simulink model "tanqueNL"  (R2018b)
settings: Solver=VariableStepAuto  StartTime=0.0  StopTime=500  RelTol=1e-3
values from neighbouring files (symbols this model uses):
  A = A    [controleLQR.m]    (also in dadosTanque.m = ssT.A; tanqueSS.m = subs(A,{qin1,qin2,h1,h2},{qin1_barra,qin2_barra,h1_barra,h2_)
  B2 = B2    [controleLQR.m]    (also in dadosTanque.m = ssT.B)
  C = C    [controleLQR.m]    (also in dadosTanque.m = ssT.C; tanqueSS.m = [1 0;0 1])
  D = D    [controleLQR.m]    (also in dadosTanque.m = ssT.D; tanqueSS.m = [0 0;0 0])
  h1 = 25    [dadosTanque.m]    (also in filterTest.m = h1_ruido(1:end-1); frequencyAnalysis.m = h1_ruido(500:1200); ssTanque.m = h1_ruido(1:end-1))
  h2 = 20    [dadosTanque.m]    (also in ssTanque.m = h2_ruido(1:end-1))
  k1 = 25    [dadosTanque.m]    (also in tanqueSS.m)
  k2 = 25    [dadosTanque.m]    (also in tanqueSS.m)
  kac = 20    [dadosTanque.m]    (also in tanqueSS.m)
  qin1 = k1*sqrt(h1) + kac*sqrt(h1-h2)    [dadosTanque.m]    (also in dados_tanque.mat = [169.72135955 169.72135955 169.72135955 169.72135955 169.721)
  qin2 = k2*sqrt(h2) - kac*sqrt(h1-h2)    [dadosTanque.m]    (also in dados_tanque.mat = [67.082039325 67.082039325 67.082039325 67.082039325 67.0820)
  stepTime = 0    [comparacao_controle_graficos.m]    (also in comparacao_sistema_graficos.m = 20; dadosTanque.m = 100)
  stepValueh1 = 1    [comparacao_controle_graficos.m]    (also in comparacao_sistema_graficos.m; dadosTanque.m)
settings Model: Creator=Caléo  LastModifiedBy=Caléo

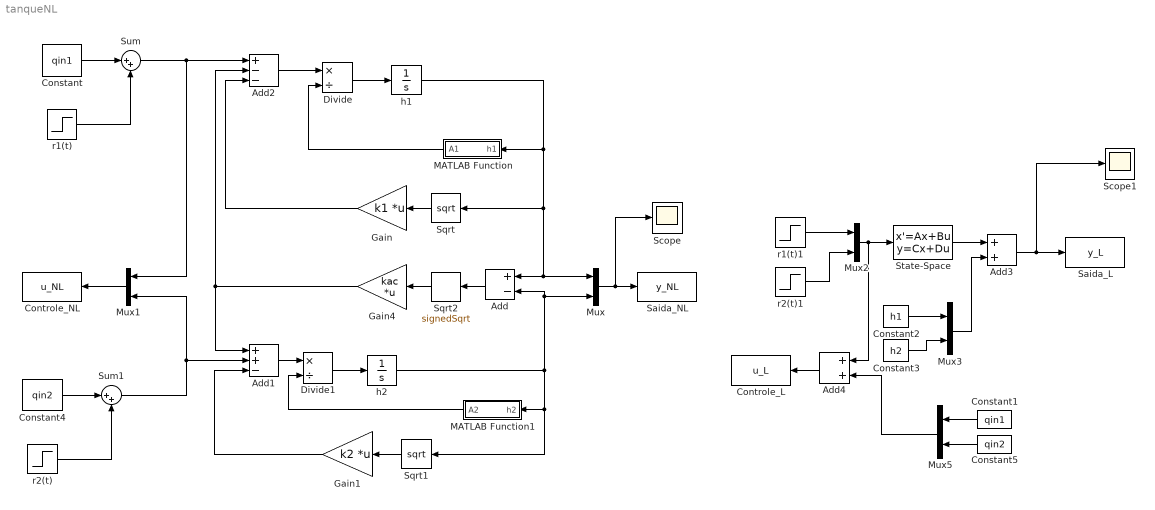
== system tanqueNL ==
  Add : Sum  Inputs=+-
  Add1 : Sum  Inputs=++-
  Add2 : Sum  Inputs=+--
  Add3 : Sum
  Add4 : Sum
  Constant : Constant  Value=qin1
  Constant1 : Constant  Value=qin1
  Constant2 : Constant  Value=h1
  Constant3 : Constant  Value=h2
  Constant4 : Constant  Value=qin2
  Constant5 : Constant  Value=qin2
  Controle_L : ToWorkspace  VariableName=u_L  SaveFormat=Timeseries  SampleTime=-1
  Controle_NL : ToWorkspace  VariableName=u_NL  SaveFormat=Timeseries  SampleTime=-1
  Divide : Product  Inputs=*/
  Divide1 : Product  Inputs=*/
  Gain : Gain  Gain=k1  Multiplication=Matrix(K*u)
  Gain1 : Gain  Gain=k2  Multiplication=Matrix(K*u)
  Gain4 : Gain  Gain=kac  Multiplication=Matrix(K*u)
  MATLAB Function : MATLAB Function  TreatAsAtomicUnit=on
  MATLAB Function1 : MATLAB Function  TreatAsAtomicUnit=on
  Mux{,1..3,5} (5 alike) : Mux  Inputs=2
  Saida_L : ToWorkspace  VariableName=y_L  SaveFormat=Timeseries  SampleTime=-1
  Saida_NL : ToWorkspace  VariableName=y_NL  SaveFormat=Timeseries  SampleTime=-1
  Scope : Scope
  Scope1 : Scope
  Sqrt : Sqrt  SaturateOnIntegerOverflow=on
  Sqrt1 : Sqrt  SaturateOnIntegerOverflow=on
  Sqrt2 : Sqrt  Operator=signedSqrt  SaturateOnIntegerOverflow=on
  State-Space : StateSpace  A=A  B=B2  C=C  D=D  InitialCondition=0
  Sum : Sum  Inputs=|++
  Sum1 : Sum  Inputs=|++
  h1 : Integrator  InitialCondition=h1  LimitOutput=on  UpperSaturationLimit=50  LowerSaturationLimit=0
  h2 : Integrator  InitialCondition=h2  LimitOutput=on  UpperSaturationLimit=50  LowerSaturationLimit=0
  r1(t) : Step  Time=stepTime  After=stepValueh1  SampleTime=0
  r1(t)1 : Step  Time=stepTime  After=stepValueh1  SampleTime=0
  r2(t) : Step  Time=stepTime  After=stepValueh1  SampleTime=0
  r2(t)1 : Step  Time=stepTime  After=stepValueh1  SampleTime=0
  wires:
  Sqrt/1 -> Gain/1
  Sqrt1/1 -> Gain1/1
  h2/1 -> Add/2, Mux/2, MATLAB Function1/1(h2), Sqrt1/1
  Add/1 -> Sqrt2/1
  Sqrt2/1 -> Gain4/1
  Gain1/1 -> Add1/3
  Gain4/1 -> Add2/2, Add1/1
  Sum1/1 -> Mux1/2, Add1/2
  Sum/1 -> Mux1/1, Add2/1
  Gain/1 -> Add2/3
  Divide/1 -> h1/1
  Mux/1 -> Scope/1, Saida_NL/1
  Mux1/1 -> Controle_NL/1
  Add2/1 -> Divide/1
  MATLAB Function/1(A1) -> Divide/2
  h1/1 -> Mux/1, Add/1, Sqrt/1, MATLAB Function/1(h1)
  Add1/1 -> Divide1/1
  Divide1/1 -> h2/1
  MATLAB Function1/1(A2) -> Divide1/2
  Mux2/1 -> State-Space/1, Add4/1
  r1(t)1/1 -> Mux2/1
  r2(t)1/1 -> Mux2/2
  Constant2/1 -> Mux3/1
  Constant3/1 -> Mux3/2
  State-Space/1 -> Add3/1
  Mux3/1 -> Add3/2
  Add3/1 -> Scope1/1, Saida_L/1
  Constant/1 -> Sum/1
  r1(t)/1 -> Sum/2
  r2(t)/1 -> Sum1/2
  Constant4/1 -> Sum1/1
  Constant1/1 -> Mux5/1
  Constant5/1 -> Mux5/2
  Mux5/1 -> Add4/2
  Add4/1 -> Controle_L/1

== matlab function tanqueNL/MATLAB Function1 ==
  data: h2 input; A2 output
function A2 = secao_tanque(h2)

    if h2 < 7.5
        d2 = 6; 
    elseif h2 < 19.5
        d2 = (19.5 - h2)/2;
    elseif h2 < 29.5
        d2 = 0;
    elseif h2 < 41.5
        d2=(h2 - 29.5)/2;
    elseif h2 >= 41.5
        d2 = 6;
    else 
        d2 = 6;
    end
    A2 = 9*(14+d2);
    
end

== matlab function tanqueNL/MATLAB Function ==
  data: h1 input; A1 output
function A1 = secao_tanque(h1)

    if h1 < 7.5
        d1 = 0;
    elseif h1 < 19.5
        d1 = (h1 - 7.5)/2;
    elseif h1 < 29.5
        d1 = 6;
    elseif h1 < 41.5
        d1 = (41.5 - h1)/2;
    elseif h1 >= 41.5
        d1 = 0;
    else 
        d1 = 0;
    end
    A1 = 9*(8+d1);
end
